simulink model "Problem2_3_3"  (R2018a)
settings: Solver=VariableStepAuto  StartTime=0.0  StopTime=100  RelTol=1e-3
settings Model: Creator=NIMA  LastModifiedBy=NIMA

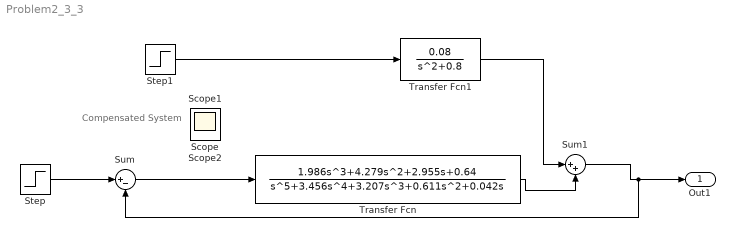
== system Problem2_3_3 ==
  note: Compensated System
  Step : Step  SampleTime=0
  Step1 : Step  Time=40  SampleTime=0
  Sum : Sum  Inputs=|+-
  Sum1 : Sum  Inputs=|++
  Transfer Fcn : TransferFcn  Numerator=[1.986 4.279 2.955 0.64]  Denominator=[1 3.456 3.207 0.611 0.042 0]
  Transfer Fcn1 : TransferFcn  Numerator=[0.08]  Denominator=[1 0 0.8]
  Out1 : Outport
  Scope : Scope
  Scope1 : Scope
  Scope2 : Scope
  wires:
  Step/1 -> Sum/1
  Sum/1 -> Transfer Fcn/1
  Transfer Fcn/1 -> Sum1/2
  Sum1/1 -> Sum/2, Out1/1
  Transfer Fcn1/1 -> Sum1/1
  Step1/1 -> Transfer Fcn1/1
